simulink model "sim"  (R2021a)
settings: Solver=VariableStepAuto  StartTime=0.0  StopTime=6  RelTol=1e-3
values from neighbouring files (symbols this model uses):
  Ka = 9.1061    [control_params.m]    (also in control_params_old.m)
  Kd1 = 0.0005399    [control_params.m]    (also in control_params_old.m; plotter.m)
  Kd2 = 1232    [control_params.m]    (also in control_params_old.m; plotter.m)
  Ki = 4.295 / (22.94 + 4.295)    (= 0.157701487057)    [control_params.m]    (also in control_params_old.m; plotter.m)
  Ko = 5    [control_params.m]    (also in control_params_old.m; plotter.m)
  Kp = 1 / (Ka * Kt * Kd1 * Kd2 * Ko * Ki)    (= 1.36850480219)    [control_params.m]
  Kp_old = 1 / (Ka * Kt)    (= 0.717754879962)    [control_params_old.m]
  Kt = 0.1530    (= 0.153)    [control_params.m]    (also in control_params_old.m)
  tau = 0.0896    [control_params.m]    (also in control_params_old.m)
  Ti = 1/z    (= 0.0827157226046)    [control_params.m]
  Ti_old = 1/z    (= 0.0827157226046)    [control_params_old.m]
undefined symbols (not defined in the file or in its folder): Kr, Kr_old
libraries: pid_lib x2
settings Model: Creator=henri  LastModifiedBy=henri

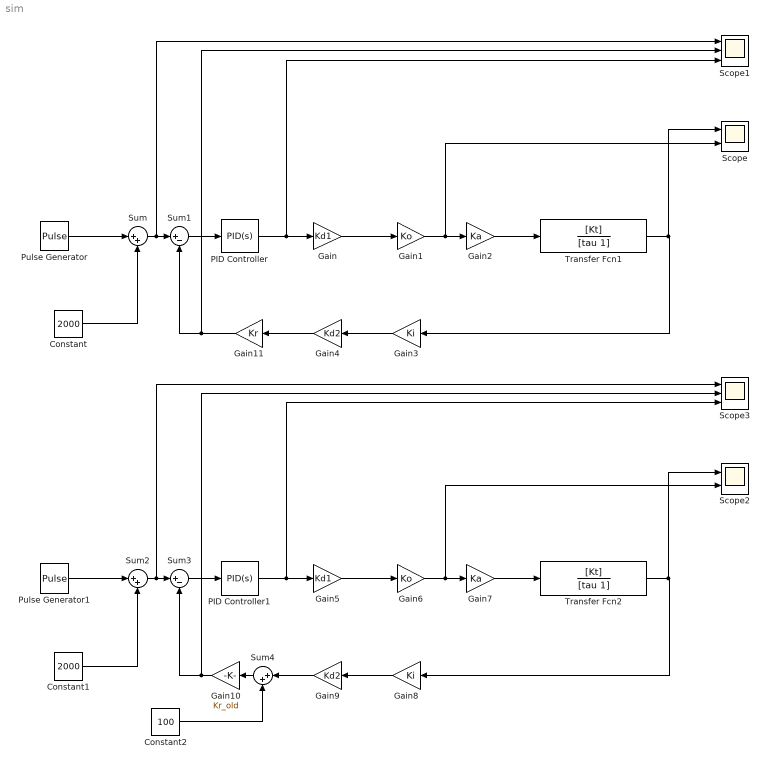
== system sim ==
  Constant : Constant  Value=2000
  Constant1 : Constant  Value=2000
  Constant2 : Constant  Value=100
  Gain : Gain  Gain=Kd1
  Gain1 : Gain  Gain=Ko
  Gain10 : Gain  Gain=Kr_old
  Gain11 : Gain  Gain=Kr
  Gain2 : Gain  Gain=Ka
  Gain3 : Gain  Gain=Ki
  Gain4 : Gain  Gain=Kd2
  Gain5 : Gain  Gain=Kd1
  Gain6 : Gain  Gain=Ko
  Gain7 : Gain  Gain=Ka
  Gain8 : Gain  Gain=Ki
  Gain9 : Gain  Gain=Kd2
  PID Controller : pid_lib/PID Controller  Controller=PID  Form=Parallel  TimeDomain=Continuous-time  UseExternalTs=off  SampleTime=-1  IntegratorMethod=Forward Euler  FilterMethod=Forward Euler  ControllerParametersSource=internal  P=Kp  I=1/Ti  D=0  UseFilter=on  N=100  TunerSelectOption=Transfer Function Based (PID Tuner App)  InitialConditionSource=internal  InitialConditionForIntegrator=0  InitialConditionForFilter=0  DifferentiatorICPrevScaledInput=0  ExternalReset=none  TrackingMode=off  Kt=1  LimitOutput=off  SatLimitsSource=internal  UpperSaturationLimit=inf  LowerSaturationLimit=-inf  LinearizeAsGain=on  AntiWindupMode=none  Kb=1  POutMin=[]  POutMax=[]  IOutMin=[]  IOutMax=[]  DOutMin=[]  DOutMax=[]  NOutMin=[]  NOutMax=[]  SumOutMin=[]  SumOutMax=[]  SaturationOutMin=[]  SaturationOutMax=[]  PParamMin=[]  PParamMax=[]  IParamMin=[]  IParamMax=[]  DParamMin=[]  DParamMax=[]  NParamMin=[]  NParamMax=[]  KbParamMin=[]  KbParamMax=[]  KtParamMin=[]  KtParamMax=[]  KbOutMin=[]  KbOutMax=[]  KtOutMin=[]  KtOutMax=[]  IntegratorOutMin=[]  IntegratorOutMax=[]  FilterOutMin=[]  FilterOutMax=[]  SumI1OutMin=[]  SumI1OutMax=[]  SumI2OutMin=[]  SumI2OutMax=[]  SumI3OutMin=[]  SumI3OutMax=[]  SumI4OutMin=[]  SumI4OutMax=[]  SumDOutMin=[]  SumDOutMax=[]  DifferentiatorOutMin=[]  DifferentiatorOutMax=[]  FilterDiffOutCoefMin=[]  FilterDiffOutCoefMax=[]  ReciprocalOutMin=[]  ReciprocalOutMax=[]  SumDenOutMin=[]  SumDenOutMax=[]  SumNumOutMin=[]  SumNumOutMax=[]  DivideOutMin=[]  DivideOutMax=[]  UdiffTsProdOutMin=[]  UdiffTsProdOutMax=[]  NTsProdOutMin=[]  NTsProdOutMax=[]  UintegralTsProdOutMin=[]  UintegralTsProdOutMax=[]  UngainTsProdOutMin=[]  UngainTsProdOutMax=[]  IntegratorContinuousStateAttributes=''  IntegratorStateMustResolveToSignalObject=off  IntegratorRTWStateStorageClass=Auto  FilterContinuousStateAttributes=''  FilterStateMustResolveToSignalObject=off  FilterRTWStateStorageClass=Auto  ParallelPVariant=InternalParameters  IdealPVariant=Disabled  IVariant=InternalParameters  DVariant=InternalParameters  IntegratorVariant=Continuous  SatVariant=Disabled  AWVariant=Passthrough  PCopyVariant=Disabled  TRVariant=Disabled  FdbkBlocksVariant=Forward  IdealPFdbkVariant=Disabled  SatFdbkVariant=Disabled  DerivativeFilterVariant=ContFilter  NVariant=InternalParameters  NCopyVariant=Disabled  FilterICVariant=InternalICsFilter  IntegratorICVariant=InternalICs  ExternalResetVariant=Disabled  TRSumVariant=Passthrough  SumFdbkVariant=Disabled  SumVariant=Sum_PID  TsampFilterVariant=InternalTs  TsampNgainVariant=Passthrough  TsampIntegralVariant=Passthrough  ExternalSaturationOutDataTypeStr=Inherit: Same as second input
  PID Controller1 : pid_lib/PID Controller  Controller=PID  Form=Parallel  TimeDomain=Continuous-time  UseExternalTs=off  SampleTime=-1  IntegratorMethod=Forward Euler  FilterMethod=Forward Euler  ControllerParametersSource=internal  P=Kp_old  I=1/Ti_old  D=0  UseFilter=on  N=100  TunerSelectOption=Transfer Function Based (PID Tuner App)  InitialConditionSource=internal  InitialConditionForIntegrator=0  InitialConditionForFilter=0  DifferentiatorICPrevScaledInput=0  ExternalReset=none  TrackingMode=off  Kt=1  LimitOutput=off  SatLimitsSource=internal  UpperSaturationLimit=inf  LowerSaturationLimit=-inf  LinearizeAsGain=on  AntiWindupMode=none  Kb=1  POutMin=[]  POutMax=[]  IOutMin=[]  IOutMax=[]  DOutMin=[]  DOutMax=[]  NOutMin=[]  NOutMax=[]  SumOutMin=[]  SumOutMax=[]  SaturationOutMin=[]  SaturationOutMax=[]  PParamMin=[]  PParamMax=[]  IParamMin=[]  IParamMax=[]  DParamMin=[]  DParamMax=[]  NParamMin=[]  NParamMax=[]  KbParamMin=[]  KbParamMax=[]  KtParamMin=[]  KtParamMax=[]  KbOutMin=[]  KbOutMax=[]  KtOutMin=[]  KtOutMax=[]  IntegratorOutMin=[]  IntegratorOutMax=[]  FilterOutMin=[]  FilterOutMax=[]  SumI1OutMin=[]  SumI1OutMax=[]  SumI2OutMin=[]  SumI2OutMax=[]  SumI3OutMin=[]  SumI3OutMax=[]  SumI4OutMin=[]  SumI4OutMax=[]  SumDOutMin=[]  SumDOutMax=[]  DifferentiatorOutMin=[]  DifferentiatorOutMax=[]  FilterDiffOutCoefMin=[]  FilterDiffOutCoefMax=[]  ReciprocalOutMin=[]  ReciprocalOutMax=[]  SumDenOutMin=[]  SumDenOutMax=[]  SumNumOutMin=[]  SumNumOutMax=[]  DivideOutMin=[]  DivideOutMax=[]  UdiffTsProdOutMin=[]  UdiffTsProdOutMax=[]  NTsProdOutMin=[]  NTsProdOutMax=[]  UintegralTsProdOutMin=[]  UintegralTsProdOutMax=[]  UngainTsProdOutMin=[]  UngainTsProdOutMax=[]  IntegratorContinuousStateAttributes=''  IntegratorStateMustResolveToSignalObject=off  IntegratorRTWStateStorageClass=Auto  FilterContinuousStateAttributes=''  FilterStateMustResolveToSignalObject=off  FilterRTWStateStorageClass=Auto  ParallelPVariant=InternalParameters  IdealPVariant=Disabled  IVariant=InternalParameters  DVariant=InternalParameters  IntegratorVariant=Continuous  SatVariant=Disabled  AWVariant=Passthrough  PCopyVariant=Disabled  TRVariant=Disabled  FdbkBlocksVariant=Forward  IdealPFdbkVariant=Disabled  SatFdbkVariant=Disabled  DerivativeFilterVariant=ContFilter  NVariant=InternalParameters  NCopyVariant=Disabled  FilterICVariant=InternalICsFilter  IntegratorICVariant=InternalICs  ExternalResetVariant=Disabled  TRSumVariant=Passthrough  SumFdbkVariant=Disabled  SumVariant=Sum_PID  TsampFilterVariant=InternalTs  TsampNgainVariant=Passthrough  TsampIntegralVariant=Passthrough  ExternalSaturationOutDataTypeStr=Inherit: Same as second input
  Pulse Generator : DiscretePulseGenerator  PulseType=Time based  Amplitude=2000  Period=3  PulseWidth=50
  Pulse Generator1 : DiscretePulseGenerator  PulseType=Time based  Amplitude=2500  Period=3  PulseWidth=50
  Scope : Scope  NumInputPorts=2
  Scope1 : Scope  NumInputPorts=3
  Scope2 : Scope  NumInputPorts=2
  Scope3 : Scope  NumInputPorts=3
  Sum : Sum  Inputs=|++
  Sum1 : Sum  Inputs=|+-
  Sum2 : Sum  Inputs=|++
  Sum3 : Sum  Inputs=|+-
  Sum4 : Sum  Inputs=|++
  Transfer Fcn1 : TransferFcn  Numerator=[Kt]  Denominator=[tau 1]
  Transfer Fcn2 : TransferFcn  Numerator=[Kt]  Denominator=[tau 1]
  wires:
  Gain/1 -> Gain1/1
  Transfer Fcn1/1 -> Scope/1, Gain3/1
  Sum4/1 -> Gain10/1
  Sum/1 -> Scope1/1, Sum1/1
  Constant2/1 -> Sum4/2
  PID Controller1/1 -> Scope3/3, Gain5/1
  Gain10/1 -> Scope3/2, Sum3/2
  Gain9/1 -> Sum4/1
  Transfer Fcn2/1 -> Scope2/1, Gain8/1
  Sum2/1 -> Scope3/1, Sum3/1
  Gain5/1 -> Gain6/1
  Gain8/1 -> Gain9/1
  Pulse Generator1/1 -> Sum2/1
  Gain7/1 -> Transfer Fcn2/1
  Gain2/1 -> Transfer Fcn1/1
  Constant1/1 -> Sum2/2
  Gain1/1 -> Scope/2, Gain2/1
  Constant/1 -> Sum/2
  Pulse Generator/1 -> Sum/1
  Sum3/1 -> PID Controller1/1
  Sum1/1 -> PID Controller/1
  Gain6/1 -> Scope2/2, Gain7/1
  Gain11/1 -> Scope1/2, Sum1/2
  Gain3/1 -> Gain4/1
  PID Controller/1 -> Scope1/3, Gain/1
  Gain4/1 -> Gain11/1
